simulink model "bamquydao"  (R2019a)
settings: Solver=VariableStepAuto  StartTime=0.0  StopTime=10  RelTol=1e-3
settings Model: Creator=dell  LastModifiedBy=dell

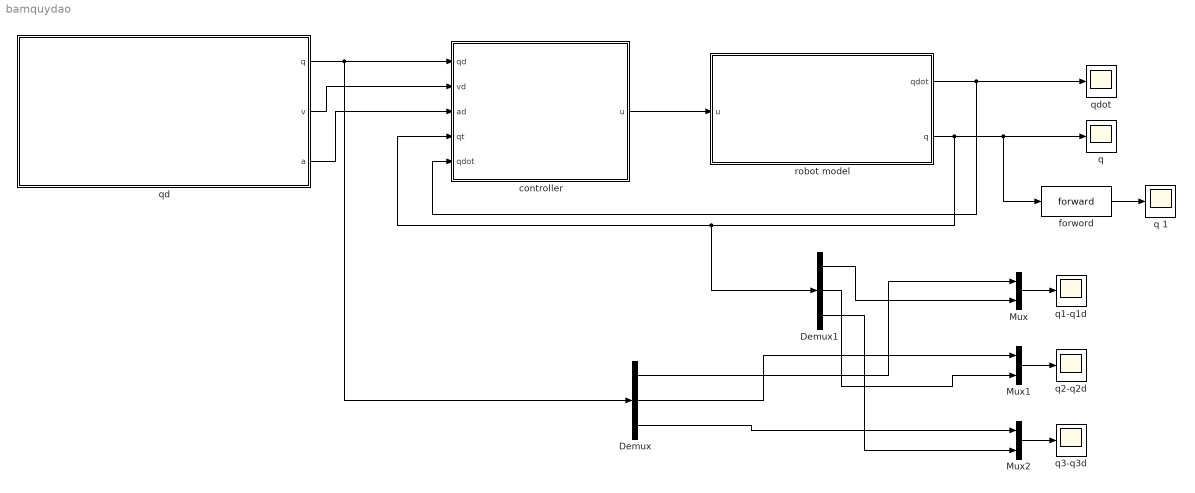
== system bamquydao ==
  Demux : Demux  Outputs=3
  Demux1 : Demux  Outputs=3
  Mux : Mux  Inputs=2
  Mux1 : Mux  Inputs=2
  Mux2 : Mux  Inputs=2
  controller : Subsystem
  forword : MATLABFcn  MATLABFcn=forward  OutputDimensions=3
  "q " : Scope
  q 1 : Scope
  q1-q1d : Scope
  q2-q2d : Scope
  q3-q3d : Scope
  qd : Subsystem
  qdot : Scope
  robot model : Subsystem
  wires:
  qd/1(q) -> Demux/1, controller/1(qd)
  robot model/2("q ") -> forword/1, "q "/1, Demux1/1, controller/4(qt)
  robot model/1(qdot) -> controller/5(qdot), qdot/1
  controller/1("u ") -> robot model/1(u)
  qd/2(v) -> controller/2(vd)
  qd/3("a ") -> controller/3(ad)
  Demux/1 -> Mux/1
  Demux1/1 -> Mux/2
  Demux/2 -> Mux1/1
  Demux1/2 -> Mux1/2
  Demux1/3 -> Mux2/2
  Demux/3 -> Mux2/1
  Mux/1 -> q1-q1d/1
  Mux1/1 -> q2-q2d/1
  Mux2/1 -> q3-q3d/1
  forword/1 -> q 1/1

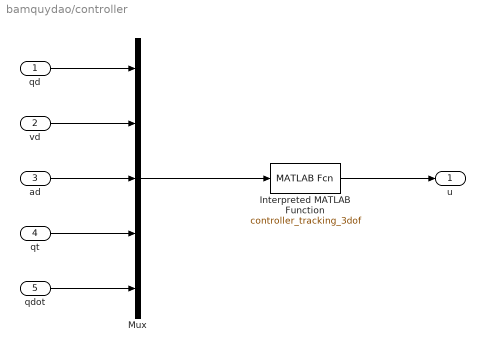
== system bamquydao/controller ==
  qd : Inport
  vd : Inport  Port=2
  ad : Inport  Port=3
  qt : Inport  Port=4
  qdot : Inport  Port=5
  Interpreted MATLAB Function : MATLABFcn  MATLABFcn=controller_tracking_3dof
  Mux : Mux  Inputs=5
  "u " : Outport
  wires:
  Mux/1 -> Interpreted MATLAB Function/1
  qd/1 -> Mux/1
  Interpreted MATLAB Function/1 -> "u "/1
  vd/1 -> Mux/2
  ad/1 -> Mux/3
  qt/1 -> Mux/4
  qdot/1 -> Mux/5

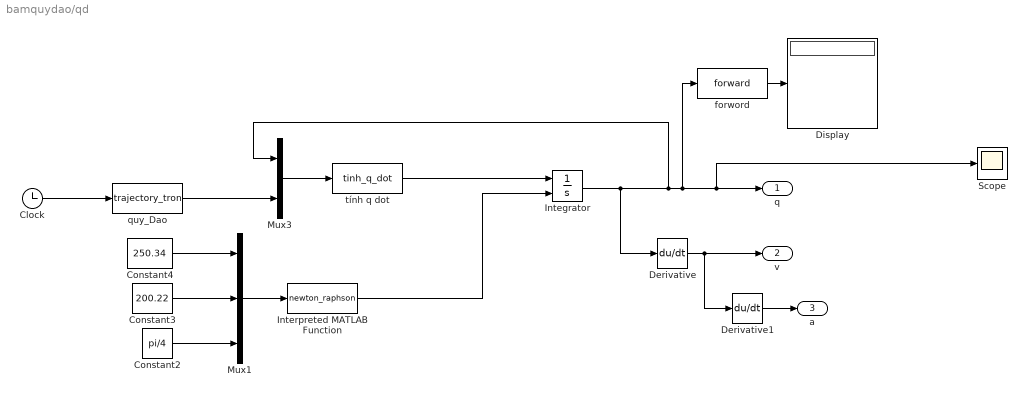
== system bamquydao/qd ==
  Clock : Clock
  Constant2 : Constant  Value=pi/4
  Constant3 : Constant  Value=200.22
  Constant4 : Constant  Value=250.34
  Derivative : Derivative
  Derivative1 : Derivative
  Display : Display
      settings: Decimation=3
  Integrator : Integrator  InitialConditionSource=external
  Interpreted MATLAB Function : MATLABFcn  MATLABFcn=newton_raphson  OutputDimensions=3
  Mux1 : Mux  Inputs=3
  Mux3 : Mux  Inputs=2
  Scope : Scope
  forword : MATLABFcn  MATLABFcn=forward  OutputDimensions=3
  quy_Dao : MATLABFcn  MATLABFcn=trajectory_tron  OutputDimensions=6
  "tính q dot " : MATLABFcn  MATLABFcn=tinh_q_dot  OutputDimensions=3
  q : Outport
  v : Outport  Port=2
  "a " : Outport  Port=3
  wires:
  Interpreted MATLAB Function/1 -> Integrator/2
  Clock/1 -> quy_Dao/1
  "tính q dot "/1 -> Integrator/1
  Integrator/1 -> Derivative/1, Mux3/1, forword/1, Scope/1, q/1
  quy_Dao/1 -> Mux3/2
  Mux3/1 -> "tính q dot "/1
  forword/1 -> Display/1
  Derivative/1 -> Derivative1/1, v/1
  Derivative1/1 -> "a "/1
  Constant4/1 -> Mux1/1
  Constant3/1 -> Mux1/2
  Constant2/1 -> Mux1/3
  Mux1/1 -> Interpreted MATLAB Function/1

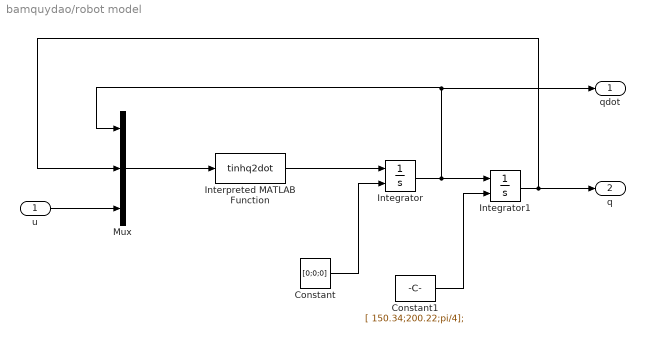
== system bamquydao/robot model ==
  u : Inport
  Constant : Constant  Value=[0;0;0]
  Constant1 : Constant  Value=[ 150.34;200.22;pi/4];
  Integrator : Integrator  InitialConditionSource=external
  Integrator1 : Integrator  InitialConditionSource=external
  Interpreted MATLAB Function : MATLABFcn  MATLABFcn=tinhq2dot
  Mux : Mux  Inputs=3
  qdot : Outport
  "q " : Outport  Port=2
  wires:
  Mux/1 -> Interpreted MATLAB Function/1
  Integrator/1 -> Mux/1, qdot/1, Integrator1/1
  u/1 -> Mux/3
  Integrator1/1 -> Mux/2, "q "/1
  Interpreted MATLAB Function/1 -> Integrator/1
  Constant/1 -> Integrator/2
  Constant1/1 -> Integrator1/2
